simulink model "robust_unstableplant_slx2020b"  (R2020b)
settings: Solver=VariableStepAuto  StartTime=0.0  StopTime=10.0  RelTol=1e-3
InitFcn:
  | idx = randi(length(Parray));
values from neighbouring files (symbols this model uses):
  Parray = stack(1,p1,p2,p3,p4,p5,p6)    [SimultaneousUnstable.m]
libraries: cstblocks x4
settings Model: Creator=philippe  LastModifiedBy=philippe

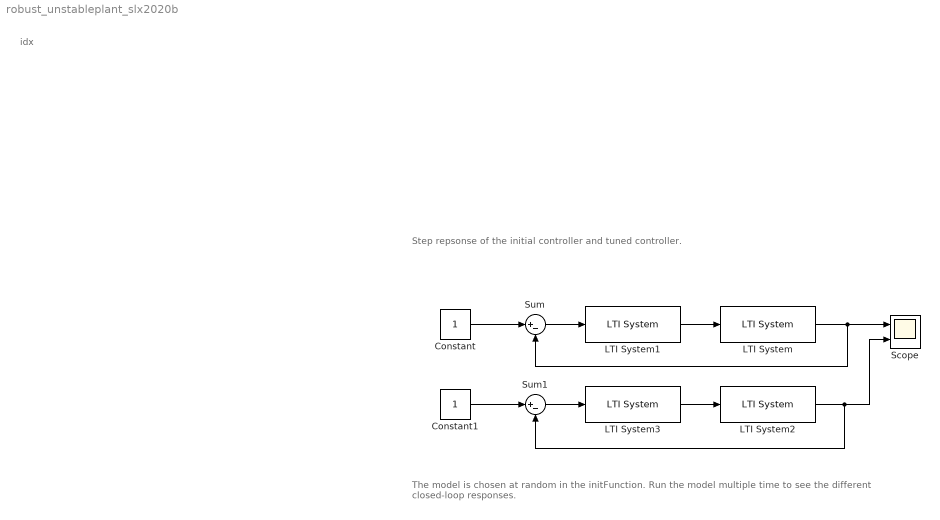
== system robust_unstableplant_slx2020b ==
  note: idx
  note: Step repsonse of the initial controller and tuned controller.
  note: The model is chosen at random in the initFunction. Run the model multiple time to see the different closed-loop responses.
  Constant : Constant
  Constant1 : Constant
  LTI System : cstblocks/LTI System  sys=Parray(:,:,idx)  IC=[]  mask(LTI Block){}
      mask Display:
      | try
      |     idx = evalin('base','idx');
      | catch
      |         idx = 0;
      | end
      | disp(sprintf('Parray(:,:,%d)',idx))
  LTI System1 : cstblocks/LTI System  sys=Kinit  IC=[]
  LTI System2 : cstblocks/LTI System  sys=Parray(:,:,idx)  IC=[]  mask(LTI Block){}
      mask Display:
      | try
      |     idx = evalin('base','idx');
      | catch
      |     idx = 0;
      | end
      | disp(sprintf('Parray(:,:,%d)',idx))
  LTI System3 : cstblocks/LTI System  sys=FB  IC=[]
  Scope : Scope  NumInputPorts=2
  Sum : Sum  Inputs=|+-
  Sum1 : Sum  Inputs=|+-
  wires:
  LTI System1/1 -> LTI System/1
  Sum/1 -> LTI System1/1
  LTI System/1 -> Sum/2, Scope/1
  Constant/1 -> Sum/1
  Sum1/1 -> LTI System3/1
  Constant1/1 -> Sum1/1
  LTI System3/1 -> LTI System2/1
  LTI System2/1 -> Scope/2, Sum1/2
